simulink model "MatlabBlueprint"  (R2017a)
settings: Solver=VariableStepAuto  StartTime=0.0  StopTime=10.0  RelTol=1e-3
libraries: hdlsllib x25, simulink x1
settings Model: Creator=rafaelmosca  LastModifiedBy=rafaelmosca

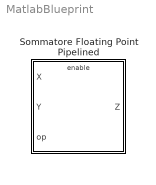
== system MatlabBlueprint ==
  Sommatore Floating Point Pipelined : Subsystem  TreatAsAtomicUnit=on

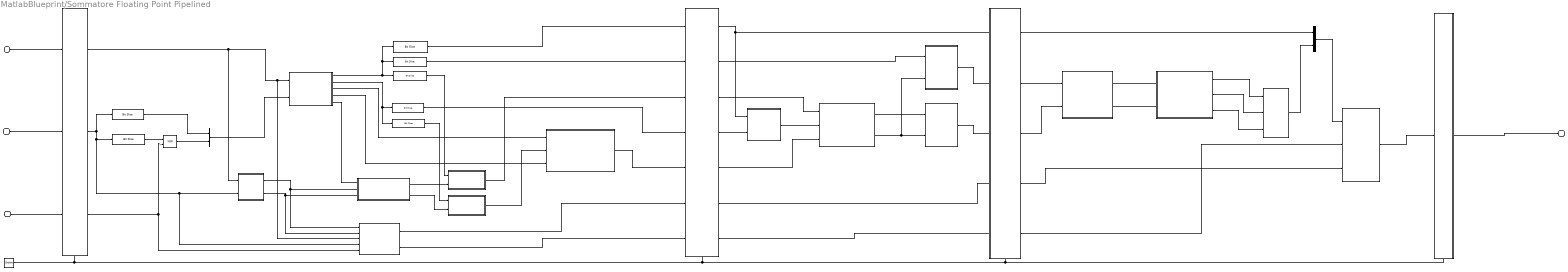
== system MatlabBlueprint/Sommatore Floating Point Pipelined ==
  note: Pre-somma
  note: Somma
  note: Correttiva
  X : Inport
  Y : Inport  Port=2
  op : Inport  Port=3
  clk : EnablePort  ShowOutputPort=on
  "Exp Adjustment " : Subsystem
  ExpChoice : Subsystem
  ExtendG : Subsystem
  ExtendS : Subsystem
  GE : hdlsllib/HDL Operations/Bit Slice  lidx=30  ridx=22
      settings: SourceProductName=HDL Coder  SourceProductBaseCode=HD
  GM : hdlsllib/HDL Operations/Bit Slice  lidx=22  ridx=0
      settings: SourceProductName=HDL Coder  SourceProductBaseCode=HD
  GS : hdlsllib/HDL Operations/Bit Slice  lidx=31  ridx=30
      settings: SourceProductName=HDL Coder  SourceProductBaseCode=HD
  MEY : hdlsllib/HDL Operations/Bit Slice  lidx=30  ridx=0
      settings: SourceProductName=HDL Coder  SourceProductBaseCode=HD
  MUX : Subsystem
  MUX Ris : Subsystem
  "Mantissa Adjustment " : Subsystem
  Normalization Module : Subsystem
  OPlogic : Subsystem
  REG1 : Subsystem  TreatAsAtomicUnit=on
  REG2 : Subsystem  TreatAsAtomicUnit=on
  REGIN : Subsystem  TreatAsAtomicUnit=on
  REGOut : Subsystem  TreatAsAtomicUnit=on
  Rounding : Subsystem
  SM : hdlsllib/HDL Operations/Bit Slice  lidx=22  ridx=0
      settings: SourceProductName=HDL Coder  SourceProductBaseCode=HD
  SS : hdlsllib/HDL Operations/Bit Slice  lidx=31  ridx=30
      settings: SourceProductName=HDL Coder  SourceProductBaseCode=HD
  SY : hdlsllib/HDL Operations/Bit Slice  lidx=31  ridx=30
      settings: SourceProductName=HDL Coder  SourceProductBaseCode=HD
  Shifter : Subsystem
  Somma Mantisse : Subsystem
  "Special Case Handler " : Subsystem
  Special Case Identifier : Subsystem
  Substraction Handling : Concatenate
  Swap : Subsystem  TreatAsAtomicUnit=on
  Vector Concatenate : Concatenate
  XOR : Logic  Operator=XOR  IconShape=distinctive  AllPortsSameDT=off  OutDataTypeStr=boolean
  Z : Outport
  wires:
  X/1 -> REGIN/1(Xin)
  Y/1 -> REGIN/2(Yin)
  clk/1 -> REGIN/Enable, REGOut/Enable, REG2/Enable, REG1/Enable
  op/1 -> REGIN/3(opin)
  REGIN/1(Xout) -> Special Case Identifier/1(X), "Special Case Handler "/3(X), Swap/1(X)
  REGIN/3("opOut ") -> XOR/2, "Special Case Handler "/5(op)
  REG1/7(isSROut) -> REG2/5(isSRin)
  MUX Ris/1(Result) -> REGOut/1(Zin)
  "Special Case Handler "/1(SpecialResult) -> REG1/6("SRin ")
  REGIN/2(Yout) -> MEY/1, SY/1, "Special Case Handler "/4(Y), Special Case Identifier/2(Y)
  GM/1 -> ExtendG/1(MG)
  Swap/1(GreatestNum) -> GS/1, GE/1, GM/1
  Swap/2(SmallestNum) -> SM/1, SS/1
  SM/1 -> ExtendS/1(MS)
  MUX/2(isSSubnormal) -> ExtendS/2(isSSubnormal)
  MUX/1(isGSubnormal) -> ExtendG/2(isGSubnormalG)
  Swap/5(swapped) -> MUX/1(Swapped)
  ExtendS/1("MSE(27) ") -> Shifter/2(Mantissa (27))
  Swap/3(Diff(5)) -> Shifter/1("ShiftNum (5) ")
  ExtendG/1("MGE(27) ") -> REG1/3(GEM)
  GE/1 -> REG1/2(GE)
  GS/1 -> REG1/1(GS)
  SS/1 -> REG1/4(SS)
  Shifter/1(Mantissa Shiftata (27)) -> REG1/5(SEM)
  REG1/3(GEMOut) -> Somma Mantisse/1("G ")
  REG1/5(SEMOut) -> Somma Mantisse/3(S)
  OPlogic/1(AdderOp) -> Somma Mantisse/2(Op)
  REG1/1(GSout) -> OPlogic/1("Segno 1 "), REG2/1(ZS)
  REG1/4(SSOut) -> OPlogic/2(Segno 2)
  REG1/6(SROut 7) -> REG2/4(SRin)
  REG2/5(isSRout) -> MUX Ris/2("isSpecialSR ")
  REG2/4(SRout 7) -> MUX Ris/3(SpecialResult)
  REG2/3(ZEMOut) -> Normalization Module/2("Mantissa ")
  REG2/2(ZEout) -> Normalization Module/1("CurrExp ")
  Normalization Module/1("NormMan ") -> Rounding/1("Mantissa ")
  Rounding/1(EsponenteCorretto(8)) -> ExpChoice/1("CurrExp ")
  Rounding/2("MantissaCorretta(23) ") -> ExpChoice/2(CurrM 1)
  ExpChoice/1(ZEM) -> Vector Concatenate/2
  REG2/1(ZSout) -> Vector Concatenate/1
  Vector Concatenate/1 -> MUX Ris/1(GenereatedResult)
  Swap/4(ForceMZero) -> Shifter/3(ForceMToZero)
  REGOut/1(Zout) -> Z/1
  SY/1 -> XOR/1
  Substraction Handling/1 -> Swap/2(Y)
  Rounding/3(isInfinity) -> ExpChoice/3(isInfinity)
  XOR/1 -> Substraction Handling/2
  MEY/1 -> Substraction Handling/1
  Special Case Identifier/2(CasoY) -> MUX/3(CaseY), "Special Case Handler "/2(CasoY)
  Special Case Identifier/1(CasoX) -> MUX/2(CaseX), "Special Case Handler "/1(CasoX)
  Somma Mantisse/2(AdditionOverflow) -> "Exp Adjustment "/2(Overflow), "Mantissa Adjustment "/2("Overflow ")
  Somma Mantisse/1("MantissaRisultato(27) ") -> "Mantissa Adjustment "/1("Mantissa ")
  "Exp Adjustment "/1(AdjExp) -> REG2/2(ZE)
  REG1/2(GEout) -> "Exp Adjustment "/1("Exp ")
  Normalization Module/2("NExp ") -> Rounding/2(Exponent)
  "Mantissa Adjustment "/1(AdjMant) -> REG2/3(ZEM)
  "Special Case Handler "/2("isSpecialResult ") -> REG1/7(isSR)

== system MatlabBlueprint/Sommatore Floating Point Pipelined/Exp Adjustment  ==
  note: Infinity
  note: Da sistemare quando è infinito
  "Exp " : Inport
  Overflow : Inport  Port=2
  Add : Sum
  Constant1 : Constant  Value=254
  Logical Operator : Logic  IconShape=distinctive  AllPortsSameDT=off  OutDataTypeStr=boolean
  Relational Operator : RelationalOperator  Operator===  OutDataTypeStr=boolean  RndMeth=Simplest
  AdjExp : Outport
  wires:
  "Exp "/1 -> Add/1, Relational Operator/2
  Constant1/1 -> Relational Operator/1
  Relational Operator/1 -> Logical Operator/1
  Overflow/1 -> Add/2, Logical Operator/2
  Logical Operator/1 -> ?
  Add/1 -> AdjExp/1

== system MatlabBlueprint/Sommatore Floating Point Pipelined/ExpChoice ==
  note: Da considerare il bit implicito e quelli di arrotondamento
  "CurrExp " : Inport
  CurrM 1 : Inport  Port=2
  isInfinity : Inport  Port=3
  ZEM : Outport

== system MatlabBlueprint/Sommatore Floating Point Pipelined/ExtendG ==
  MG : Inport
  isGSubnormalG : Inport  Port=2
  Constant : Constant  Value=000
  ImplicitBit : Logic  Operator=NOT  IconShape=distinctive  AllPortsSameDT=off  OutDataTypeStr=boolean
  Vector Concatenate : Concatenate  NumInputs=3
  "MGE(27) " : Outport
  wires:
  Vector Concatenate/1 -> "MGE(27) "/1
  isGSubnormalG/1 -> ImplicitBit/1
  ImplicitBit/1 -> Vector Concatenate/1
  MG/1 -> Vector Concatenate/2
  Constant/1 -> Vector Concatenate/3

== system MatlabBlueprint/Sommatore Floating Point Pipelined/ExtendS ==
  MS : Inport
  isSSubnormal : Inport  Port=2
  Constant : Constant  Value=000
  ImplicitBit : Logic  Operator=NOT  IconShape=distinctive  AllPortsSameDT=off  OutDataTypeStr=boolean
  Vector Concatenate : Concatenate  NumInputs=3
  "MSE(27) " : Outport
  wires:
  Vector Concatenate/1 -> "MSE(27) "/1
  isSSubnormal/1 -> ImplicitBit/1
  MS/1 -> Vector Concatenate/2
  Constant/1 -> Vector Concatenate/3
  ImplicitBit/1 -> Vector Concatenate/1

== system MatlabBlueprint/Sommatore Floating Point Pipelined/MUX ==
  note: if SWAPPED=1 CASO Y becomes CASOG
  Swapped : Inport
  CaseX : Inport  Port=2
  CaseY : Inport  Port=3
  isXSubnormal : hdlsllib/HDL Operations/Bit Slice  lidx=3  ridx=3
      settings: SourceProductName=HDL Coder  SourceProductBaseCode=HD
  isYSubnormal : hdlsllib/HDL Operations/Bit Slice  lidx=3  ridx=3
      settings: SourceProductName=HDL Coder  SourceProductBaseCode=HD
  isGSubnormal : Outport
  isSSubnormal : Outport  Port=2
  wires:
  CaseX/1 -> isXSubnormal/1
  CaseY/1 -> isYSubnormal/1

== system MatlabBlueprint/Sommatore Floating Point Pipelined/MUX Ris ==
  GenereatedResult : Inport
  "isSpecialSR " : Inport  Port=2
  SpecialResult : Inport  Port=3
  Result : Outport
  wires:
  GenereatedResult/1 -> ?

== system MatlabBlueprint/Sommatore Floating Point Pipelined/Mantissa Adjustment  ==
  note: perdo l'ultimo
  note: shift a destra di una posizione per gestire l'overflow
  note: 0
  note: 1
  "Mantissa " : Inport
  "Overflow " : Inport  Port=2
  "       " : hdlsllib/HDL Operations/Bit Slice  lidx=26  ridx=1
      settings: SourceProductName=HDL Coder  SourceProductBaseCode=HD
  Switch : Switch  Criteria=u2 ~= 0
  Vector Concatenate : Concatenate
  AdjMant : Outport
  wires:
  Switch/1 -> AdjMant/1
  "       "/1 -> Vector Concatenate/2
  "Mantissa "/1 -> Switch/1, "       "/1
  "Overflow "/1 -> Vector Concatenate/1, Switch/2
  Vector Concatenate/1 -> Switch/3

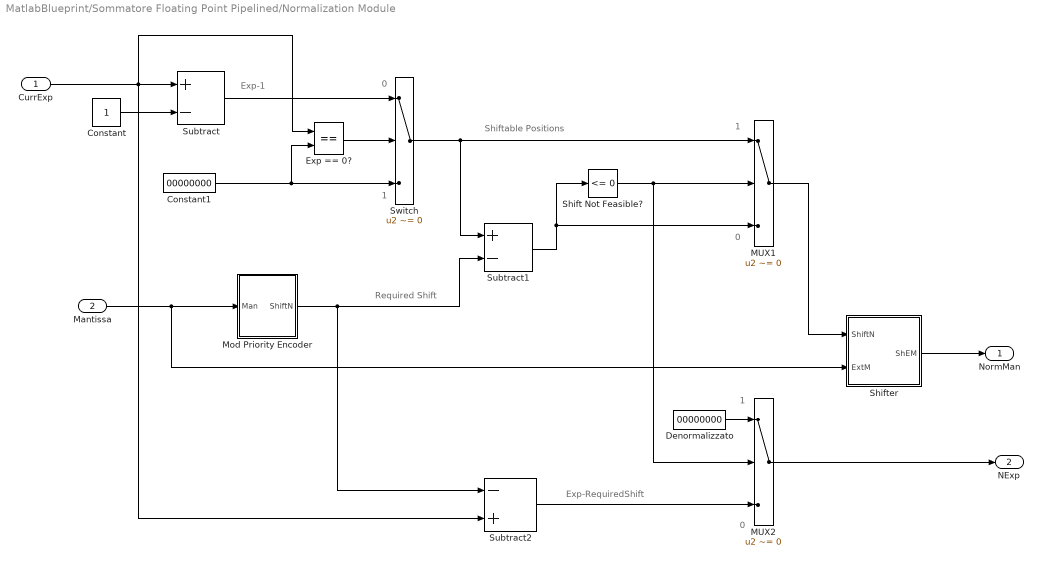
== system MatlabBlueprint/Sommatore Floating Point Pipelined/Normalization Module ==
  note: Exp-1
  note: Exp-RequiredShift
  note: Required Shift
  note: 0
  note: Shiftable Positions
  note: 1
  note: 1
  note: 0
  note: 1
  note: 0
  "CurrExp " : Inport
  "Mantissa " : Inport  Port=2
  Constant : Constant
  Constant1 : Constant  Value=00000000
  Denormalizzato : Constant  Value=00000000
  Exp == 0? : RelationalOperator  Operator===  OutDataTypeStr=boolean  RndMeth=Simplest
  MUX1 : Switch  Criteria=u2 ~= 0
  MUX2 : Switch  Criteria=u2 ~= 0
  "Mod Priority Encoder " : Subsystem
  Shift Not Feasible? : simulink/Logic and Bit Operations/Compare To Zero  relop=<=  OutDataTypeStr=boolean
  Shifter : Subsystem
  Subtract : Sum  Inputs=+-
  Subtract1 : Sum  Inputs=+-
  "Subtract2 " : Sum  Inputs=-+
  Switch : Switch  Criteria=u2 ~= 0
  "NormMan " : Outport
  "NExp " : Outport  Port=2
  wires:
  "Mantissa "/1 -> "Mod Priority Encoder "/1(Man), Shifter/2(ExtM)
  "CurrExp "/1 -> "Subtract2 "/2, Subtract/1, Exp == 0?/1
  "Mod Priority Encoder "/1(ShiftN) -> "Subtract2 "/1, Subtract1/2
  Shifter/1(ShEM) -> "NormMan "/1
  Constant/1 -> Subtract/2
  Subtract/1 -> Switch/1
  Exp == 0?/1 -> Switch/2
  Constant1/1 -> Switch/3, Exp == 0?/2
  Switch/1 -> MUX1/1, Subtract1/1
  MUX1/1 -> Shifter/1("ShiftN ")
  Subtract1/1 -> Shift Not Feasible?/1, MUX1/3
  Shift Not Feasible?/1 -> MUX2/2, MUX1/2
  "Subtract2 "/1 -> MUX2/3
  Denormalizzato/1 -> MUX2/1
  MUX2/1 -> "NExp "/1

== system MatlabBlueprint/Sommatore Floating Point Pipelined/OPlogic ==
  note: Non conta l'ordine!!!!! il segno viene gestit dal numero più grande
  "Segno 1 " : Inport
  Segno 2 : Inport  Port=2
  OpLogic : Logic  Operator=XOR  IconShape=distinctive  AllPortsSameDT=off  OutDataTypeStr=boolean
  AdderOp : Outport
  wires:
  "Segno 1 "/1 -> OpLogic/1
  Segno 2/1 -> OpLogic/2
  OpLogic/1 -> AdderOp/1

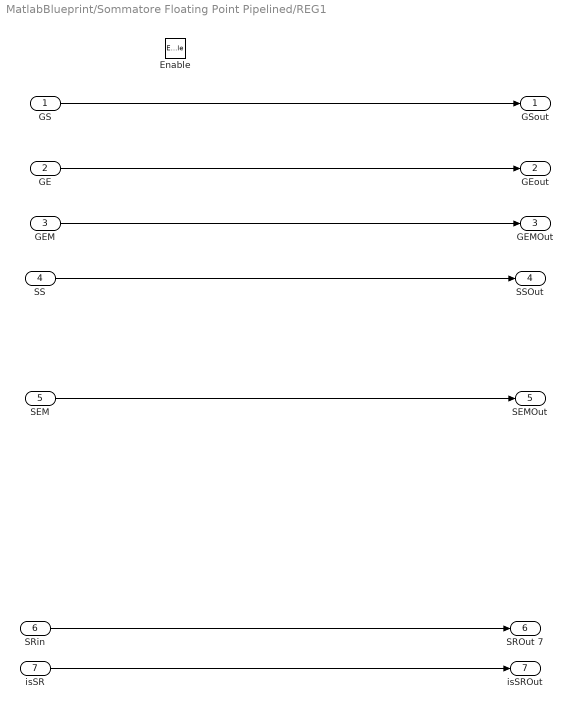
== system MatlabBlueprint/Sommatore Floating Point Pipelined/REG1 ==
  GS : Inport
  GE : Inport  Port=2
  GEM : Inport  Port=3
  SS : Inport  Port=4
  SEM : Inport  Port=5
  "SRin " : Inport  Port=6
  isSR : Inport  Port=7
  Enable : EnablePort
  GSout : Outport
  GEout : Outport  Port=2
  GEMOut : Outport  Port=3
  SSOut : Outport  Port=4
  SEMOut : Outport  Port=5
  SROut 7 : Outport  Port=6
  isSROut : Outport  Port=7
  wires:
  GS/1 -> GSout/1
  GE/1 -> GEout/1
  GEM/1 -> GEMOut/1
  SS/1 -> SSOut/1
  SEM/1 -> SEMOut/1
  "SRin "/1 -> SROut 7/1
  isSR/1 -> isSROut/1

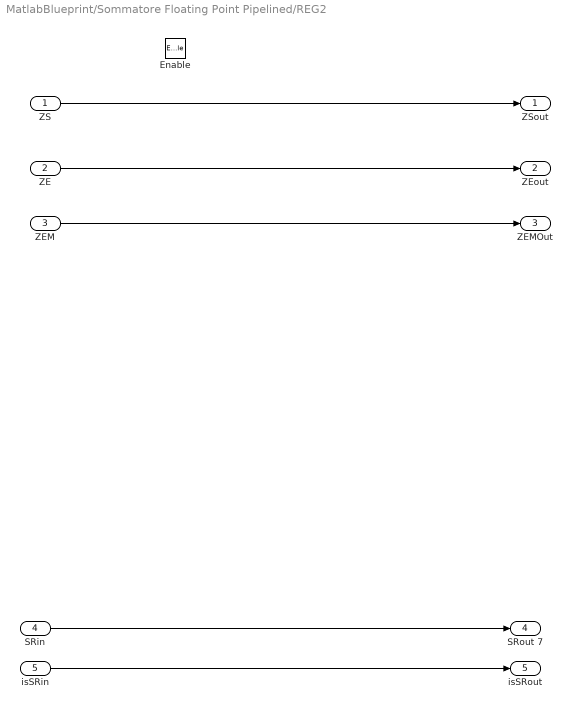
== system MatlabBlueprint/Sommatore Floating Point Pipelined/REG2 ==
  ZS : Inport
  ZE : Inport  Port=2
  ZEM : Inport  Port=3
  SRin : Inport  Port=4
  isSRin : Inport  Port=5
  Enable : EnablePort
  ZSout : Outport
  ZEout : Outport  Port=2
  ZEMOut : Outport  Port=3
  SRout 7 : Outport  Port=4
  isSRout : Outport  Port=5
  wires:
  ZS/1 -> ZSout/1
  ZE/1 -> ZEout/1
  ZEM/1 -> ZEMOut/1
  SRin/1 -> SRout 7/1
  isSRin/1 -> isSRout/1

== system MatlabBlueprint/Sommatore Floating Point Pipelined/REGIN ==
  Xin : Inport
  Yin : Inport  Port=2
  opin : Inport  Port=3
  Enable : EnablePort
  Xout : Outport
  Yout : Outport  Port=2
  "opOut " : Outport  Port=3
  wires:
  Xin/1 -> Xout/1
  Yin/1 -> Yout/1
  opin/1 -> "opOut "/1

== system MatlabBlueprint/Sommatore Floating Point Pipelined/REGOut ==
  Zin : Inport
  Enable : EnablePort
  Zout : Outport
  wires:
  Zin/1 -> Zout/1

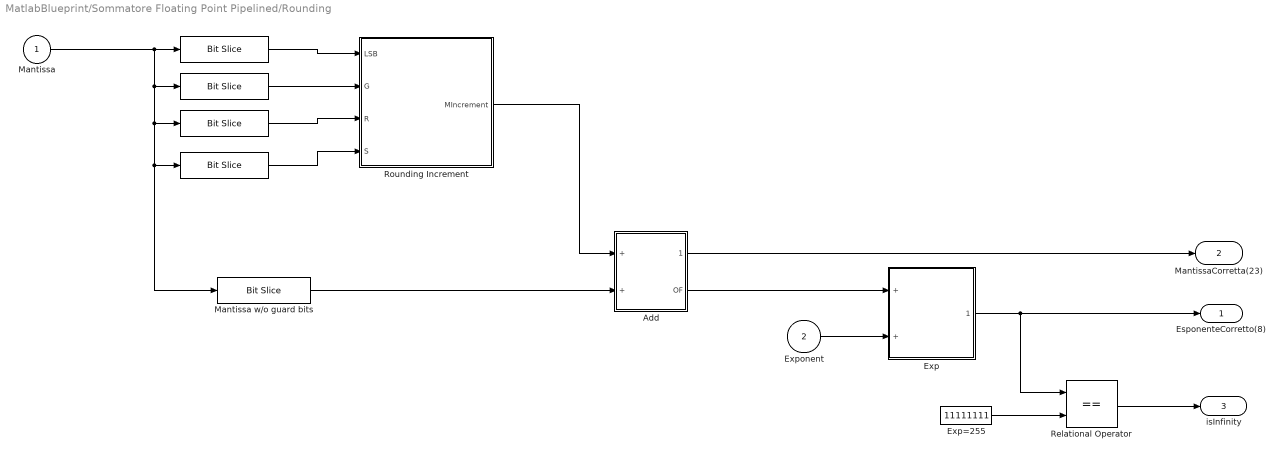
== system MatlabBlueprint/Sommatore Floating Point Pipelined/Rounding ==
  "Mantissa " : Inport
  Exponent : Inport  Port=2
  " " : hdlsllib/HDL Operations/Bit Slice  lidx=3  ridx=3
      settings: SourceProductName=HDL Coder  SourceProductBaseCode=HD
  "  " : hdlsllib/HDL Operations/Bit Slice  lidx=0  ridx=0
      settings: SourceProductName=HDL Coder  SourceProductBaseCode=HD
  "   " : hdlsllib/HDL Operations/Bit Slice  lidx=2  ridx=2
      settings: SourceProductName=HDL Coder  SourceProductBaseCode=HD
  "       " : hdlsllib/HDL Operations/Bit Slice  lidx=1  ridx=1
      settings: SourceProductName=HDL Coder  SourceProductBaseCode=HD
  "  Mantissa w/o guard bits" : hdlsllib/HDL Operations/Bit Slice  lidx=25  ridx=3
      settings: SourceProductName=HDL Coder  SourceProductBaseCode=HD
  Add : Subsystem
  Exp : Subsystem
  Exp=255 : Constant  Value=11111111
  Relational Operator : RelationalOperator  Operator===  OutDataTypeStr=boolean  RndMeth=Simplest
  Rounding Increment : Subsystem
  EsponenteCorretto(8) : Outport
  "MantissaCorretta(23) " : Outport  Port=2
  isInfinity : Outport  Port=3
  wires:
  "Mantissa "/1 -> "  Mantissa w/o guard bits"/1, "  "/1, "       "/1, "   "/1, " "/1
  " "/1 -> Rounding Increment/1("LSB ")
  "   "/1 -> Rounding Increment/2("G ")
  "       "/1 -> Rounding Increment/3(R)
  "  "/1 -> Rounding Increment/4(S)
  Rounding Increment/1("MIncrement ") -> Add/1("+ ")
  "  Mantissa w/o guard bits"/1 -> Add/2("+ ")
  Add/2(" OF") -> Exp/1("+ ")
  Exponent/1 -> Exp/2("+ ")
  Add/1(" ") -> "MantissaCorretta(23) "/1
  Exp/1(" ") -> EsponenteCorretto(8)/1, Relational Operator/1
  Relational Operator/1 -> isInfinity/1
  Exp=255/1 -> Relational Operator/2

== system MatlabBlueprint/Sommatore Floating Point Pipelined/Shifter ==
  "ShiftNum (5) " : Inport
  Mantissa (27) : Inport  Port=2
  ForceMToZero : Inport  Port=3
  Esempio 4 bit : Subsystem
  Mantissa Shiftata (27) : Outport

== system MatlabBlueprint/Sommatore Floating Point Pipelined/Somma Mantisse ==
  note: Da considerare il bit implicito e quelli di arrotondamento
  "G " : Inport
  Op : Inport  Port=2
  S : Inport  Port=3
  "MantissaRisultato(27) " : Outport
  AdditionOverflow : Outport  Port=2

== system MatlabBlueprint/Sommatore Floating Point Pipelined/Special Case Handler  ==
  CasoX : Inport
  CasoY : Inport  Port=2
  X : Inport  Port=3
  Y : Inport  Port=4
  op : Inport  Port=5
  SpecialResult : Outport
  "isSpecialResult " : Outport  Port=2

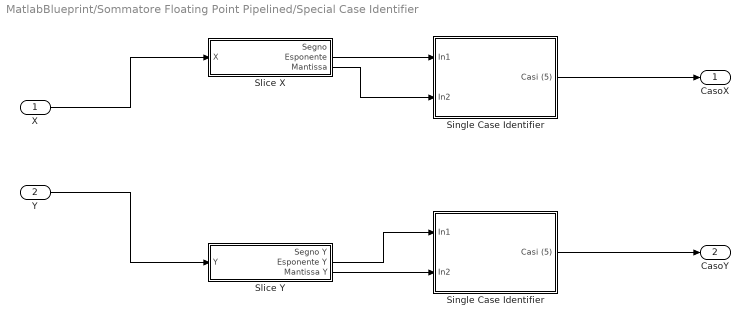
== system MatlabBlueprint/Sommatore Floating Point Pipelined/Special Case Identifier ==
  X : Inport
  Y : Inport  Port=2
  Single Case Identifier : Subsystem
  "Single Case Identifier " : Subsystem
  Slice X : Subsystem
  Slice Y : Subsystem
  CasoX : Outport
  CasoY : Outport  Port=2
  wires:
  Slice Y/3(Mantissa Y) -> "Single Case Identifier "/2(In2)
  Slice X/3(Mantissa) -> Single Case Identifier/2(In2)
  Slice Y/2(Esponente Y) -> "Single Case Identifier "/1(In1)
  Slice X/2(Esponente) -> Single Case Identifier/1(In1)
  X/1 -> Slice X/1("X ")
  Y/1 -> Slice Y/1("Y ")
  Single Case Identifier/1(Casi (5)) -> CasoX/1
  "Single Case Identifier "/1(Casi (5)) -> CasoY/1

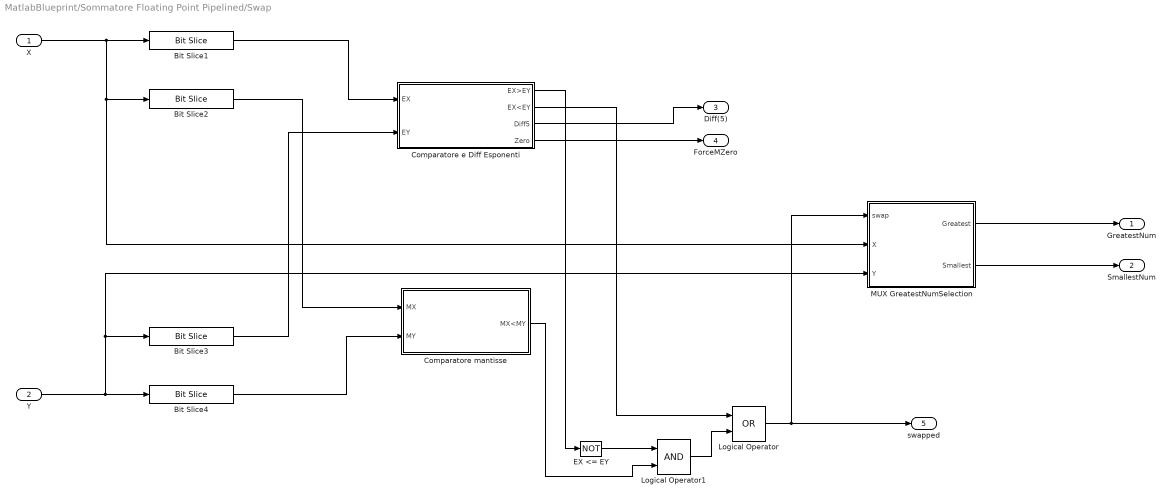
== system MatlabBlueprint/Sommatore Floating Point Pipelined/Swap ==
  X : Inport
  Y : Inport  Port=2
  Bit Slice1 : hdlsllib/HDL Operations/Bit Slice  lidx=30  ridx=22
      settings: SourceProductName=HDL Coder  SourceProductBaseCode=HD
  Bit Slice2 : hdlsllib/HDL Operations/Bit Slice  lidx=22  ridx=0
      settings: SourceProductName=HDL Coder  SourceProductBaseCode=HD
  Bit Slice3 : hdlsllib/HDL Operations/Bit Slice  lidx=30  ridx=22
      settings: SourceProductName=HDL Coder  SourceProductBaseCode=HD
  Bit Slice4 : hdlsllib/HDL Operations/Bit Slice  lidx=22  ridx=0
      settings: SourceProductName=HDL Coder  SourceProductBaseCode=HD
  Comparatore e Diff Esponenti : Subsystem
  Comparatore mantisse : Subsystem
  EX <= EY : Logic  Operator=NOT  IconShape=distinctive  AllPortsSameDT=off  OutDataTypeStr=boolean
  Logical Operator : Logic  Operator=OR  IconShape=distinctive  AllPortsSameDT=off  OutDataTypeStr=boolean
  Logical Operator1 : Logic  IconShape=distinctive  AllPortsSameDT=off  OutDataTypeStr=boolean
  MUX GreatestNumSelection : Subsystem
  GreatestNum : Outport
  SmallestNum : Outport  Port=2
  Diff(5) : Outport  Port=3
  ForceMZero : Outport  Port=4
  swapped : Outport  Port=5
  wires:
  Y/1 -> Bit Slice4/1, MUX GreatestNumSelection/3(Y), Bit Slice3/1
  Bit Slice1/1 -> Comparatore e Diff Esponenti/1(EX)
  Bit Slice3/1 -> Comparatore e Diff Esponenti/2(EY)
  Bit Slice2/1 -> Comparatore mantisse/1(MX)
  Bit Slice4/1 -> Comparatore mantisse/2(MY)
  Comparatore e Diff Esponenti/1(EX>EY) -> EX <= EY/1
  MUX GreatestNumSelection/2("Smallest ") -> SmallestNum/1
  Logical Operator1/1 -> Logical Operator/2
  Logical Operator/1 -> swapped/1, MUX GreatestNumSelection/1("swap ")
  X/1 -> Bit Slice1/1, MUX GreatestNumSelection/2(X), Bit Slice2/1
  Comparatore e Diff Esponenti/2(EX<EY) -> Logical Operator/1
  Comparatore mantisse/1(MX<MY) -> Logical Operator1/2
  EX <= EY/1 -> Logical Operator1/1
  MUX GreatestNumSelection/1(Greatest) -> GreatestNum/1
  Comparatore e Diff Esponenti/3(Diff5) -> Diff(5)/1
  Comparatore e Diff Esponenti/4(Zero) -> ForceMZero/1

== system MatlabBlueprint/Sommatore Floating Point Pipelined/Normalization Module/Mod Priority Encoder  ==
  note: 5 bit
  Man : Inport
  ShiftN : Outport

== system MatlabBlueprint/Sommatore Floating Point Pipelined/Normalization Module/Shifter ==
  "ShiftN " : Inport
  ExtM : Inport  Port=2
  ShEM : Outport

== system MatlabBlueprint/Sommatore Floating Point Pipelined/Rounding/Add ==
  "+ " : Inport
  "+ " : Inport  Port=2
  " " : Outport
  " OF" : Outport  Port=2

== system MatlabBlueprint/Sommatore Floating Point Pipelined/Rounding/Exp ==
  "+ " : Inport
  "+ " : Inport  Port=2
  " " : Outport

== system MatlabBlueprint/Sommatore Floating Point Pipelined/Rounding/Rounding Increment ==
  "LSB " : Inport
  "G " : Inport  Port=2
  R : Inport  Port=3
  S : Inport  Port=4
  "MIncrement " : Outport

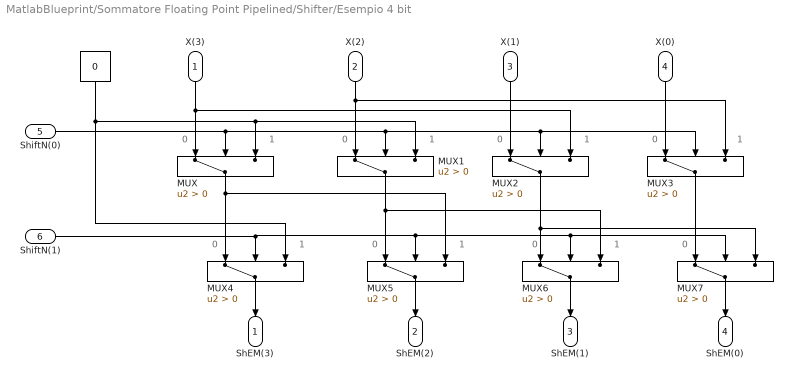
== system MatlabBlueprint/Sommatore Floating Point Pipelined/Shifter/Esempio 4 bit ==
  note: 0
  note: 1
  note: 1
  note: 0
  note: 0
  note: 0
  note: 0
  note: 1
  note: 0
  note: 1
  note: 1
  note: 1
  note: 0
  note: 0
  note: 1
  X(3) : Inport
  X(2) : Inport  Port=2
  X(1) : Inport  Port=3
  X(0) : Inport  Port=4
  ShiftN(0) : Inport  Port=5
  ShiftN(1) : Inport  Port=6
  " " : Constant  Value=0
  MUX{,1..7} (8 alike) : Switch  Criteria=u2 > Threshold
  ShEM(3) : Outport
  ShEM(2) : Outport  Port=2
  ShEM(1) : Outport  Port=3
  ShEM(0) : Outport  Port=4
  wires:
  MUX2/1 -> MUX7/3, MUX6/1
  X(1)/1 -> MUX2/1
  ShiftN(0)/1 -> MUX/2, MUX1/2, MUX2/2, MUX3/2
  X(2)/1 -> MUX1/1, MUX3/3
  MUX/1 -> MUX4/1, MUX5/3
  " "/1 -> MUX4/3, MUX/3, MUX1/3
  MUX4/1 -> ShEM(3)/1
  MUX5/1 -> ShEM(2)/1
  X(0)/1 -> MUX3/1
  MUX3/1 -> MUX7/1
  X(3)/1 -> MUX/1, MUX2/3
  MUX6/1 -> ShEM(1)/1
  ShiftN(1)/1 -> MUX5/2, MUX6/2, MUX7/2, MUX4/2
  MUX1/1 -> MUX6/3, MUX5/1
  MUX7/1 -> ShEM(0)/1

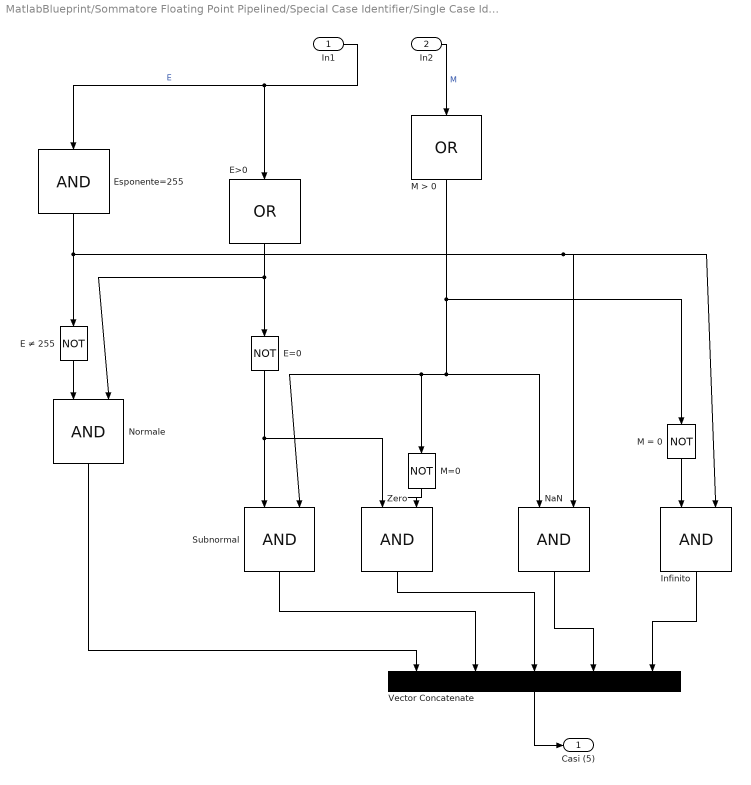
== system MatlabBlueprint/Sommatore Floating Point Pipelined/Special Case Identifier/Single Case Identifier ==
  In1 : Inport
  In2 : Inport  Port=2
  E ≠ 255 : Logic  Operator=NOT  Inputs=1  IconShape=distinctive  AllPortsSameDT=off  OutDataTypeStr=boolean
  E=0 : Logic  Operator=NOT  Inputs=1  IconShape=distinctive  AllPortsSameDT=off  OutDataTypeStr=boolean
  E>0 : Logic  Operator=OR  Inputs=1  IconShape=distinctive  AllPortsSameDT=off  OutDataTypeStr=boolean
  Esponente=255 : Logic  Inputs=1  IconShape=distinctive  AllPortsSameDT=off  OutDataTypeStr=boolean
  Infinito : Logic  IconShape=distinctive  AllPortsSameDT=off  OutDataTypeStr=boolean
  M = 0 : Logic  Operator=NOT  Inputs=1  IconShape=distinctive  AllPortsSameDT=off  OutDataTypeStr=boolean
  M > 0 : Logic  Operator=OR  Inputs=1  IconShape=distinctive  AllPortsSameDT=off  OutDataTypeStr=boolean
  M=0 : Logic  Operator=NOT  Inputs=1  IconShape=distinctive  AllPortsSameDT=off  OutDataTypeStr=boolean
  NaN : Logic  IconShape=distinctive  AllPortsSameDT=off  OutDataTypeStr=boolean
  Normale : Logic  IconShape=distinctive  AllPortsSameDT=off  OutDataTypeStr=boolean
  Subnormal : Logic  IconShape=distinctive  AllPortsSameDT=off  OutDataTypeStr=boolean
  Vector Concatenate : Concatenate  NumInputs=5
  Zero : Logic  IconShape=distinctive  AllPortsSameDT=off  OutDataTypeStr=boolean
  Casi (5) : Outport
  wires:
  Vector Concatenate/1 -> Casi (5)/1
  Normale/1 -> Vector Concatenate/1
  M = 0/1 -> Infinito/1
  NaN/1 -> Vector Concatenate/4
  M=0/1 -> Zero/2
  Subnormal/1 -> Vector Concatenate/2
  E=0/1 -> Zero/1, Subnormal/1
  In2/1 -> M > 0/1  "M"
  Infinito/1 -> Vector Concatenate/5
  E>0/1 -> Normale/2, E=0/1
  In1/1 -> E>0/1, Esponente=255/1  "E"
  M > 0/1 -> M = 0/1, NaN/1, M=0/1, Subnormal/2
  Zero/1 -> Vector Concatenate/3
  Esponente=255/1 -> E ≠ 255/1, Infinito/2, NaN/2
  E ≠ 255/1 -> Normale/1

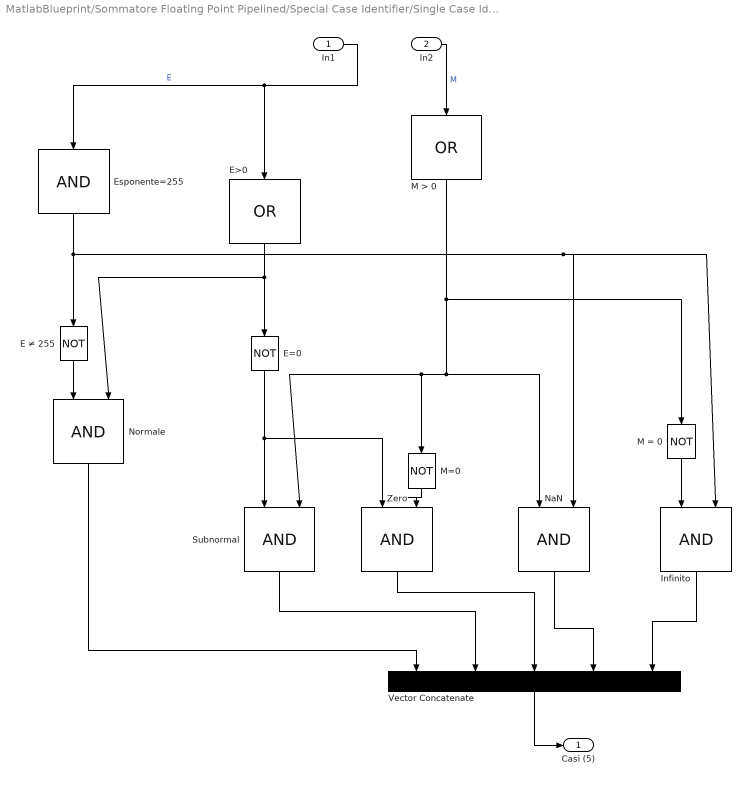
== system MatlabBlueprint/Sommatore Floating Point Pipelined/Special Case Identifier/Single Case Identifier  ==
  In1 : Inport
  In2 : Inport  Port=2
  E ≠ 255 : Logic  Operator=NOT  Inputs=1  IconShape=distinctive  AllPortsSameDT=off  OutDataTypeStr=boolean
  E=0 : Logic  Operator=NOT  Inputs=1  IconShape=distinctive  AllPortsSameDT=off  OutDataTypeStr=boolean
  E>0 : Logic  Operator=OR  Inputs=1  IconShape=distinctive  AllPortsSameDT=off  OutDataTypeStr=boolean
  Esponente=255 : Logic  Inputs=1  IconShape=distinctive  AllPortsSameDT=off  OutDataTypeStr=boolean
  Infinito : Logic  IconShape=distinctive  AllPortsSameDT=off  OutDataTypeStr=boolean
  M = 0 : Logic  Operator=NOT  Inputs=1  IconShape=distinctive  AllPortsSameDT=off  OutDataTypeStr=boolean
  M > 0 : Logic  Operator=OR  Inputs=1  IconShape=distinctive  AllPortsSameDT=off  OutDataTypeStr=boolean
  M=0 : Logic  Operator=NOT  Inputs=1  IconShape=distinctive  AllPortsSameDT=off  OutDataTypeStr=boolean
  NaN : Logic  IconShape=distinctive  AllPortsSameDT=off  OutDataTypeStr=boolean
  Normale : Logic  IconShape=distinctive  AllPortsSameDT=off  OutDataTypeStr=boolean
  Subnormal : Logic  IconShape=distinctive  AllPortsSameDT=off  OutDataTypeStr=boolean
  Vector Concatenate : Concatenate  NumInputs=5
  Zero : Logic  IconShape=distinctive  AllPortsSameDT=off  OutDataTypeStr=boolean
  Casi (5) : Outport
  wires:
  E>0/1 -> Normale/2, E=0/1
  Subnormal/1 -> Vector Concatenate/2
  NaN/1 -> Vector Concatenate/4
  E=0/1 -> Zero/1, Subnormal/1
  Normale/1 -> Vector Concatenate/1
  In2/1 -> M > 0/1  "M"
  Infinito/1 -> Vector Concatenate/5
  Vector Concatenate/1 -> Casi (5)/1
  M = 0/1 -> Infinito/1
  In1/1 -> E>0/1, Esponente=255/1  "E"
  M=0/1 -> Zero/2
  M > 0/1 -> M = 0/1, NaN/1, M=0/1, Subnormal/2
  Zero/1 -> Vector Concatenate/3
  Esponente=255/1 -> E ≠ 255/1, Infinito/2, NaN/2
  E ≠ 255/1 -> Normale/1

== system MatlabBlueprint/Sommatore Floating Point Pipelined/Special Case Identifier/Slice X ==
  "X " : Inport
  Esponente X : hdlsllib/HDL Operations/Bit Slice  lidx=30  ridx=22
      settings: SourceProductName=HDL Coder  SourceProductBaseCode=HD
  Mantissa X : hdlsllib/HDL Operations/Bit Slice  lidx=22  ridx=0
      settings: SourceProductName=HDL Coder  SourceProductBaseCode=HD
  "Segno X " : hdlsllib/HDL Operations/Bit Slice  lidx=31  ridx=30
      settings: SourceProductName=HDL Coder  SourceProductBaseCode=HD
  Segno : Outport
  Esponente : Outport  Port=2
  Mantissa : Outport  Port=3
  wires:
  "Segno X "/1 -> Segno/1
  "X "/1 -> Mantissa X/1, Esponente X/1, "Segno X "/1
  Esponente X/1 -> Esponente/1
  Mantissa X/1 -> Mantissa/1

== system MatlabBlueprint/Sommatore Floating Point Pipelined/Special Case Identifier/Slice Y ==
  "Y " : Inport
  Esponente X : hdlsllib/HDL Operations/Bit Slice  lidx=30  ridx=22
      settings: SourceProductName=HDL Coder  SourceProductBaseCode=HD
  Mantissa X : hdlsllib/HDL Operations/Bit Slice  lidx=22  ridx=0
      settings: SourceProductName=HDL Coder  SourceProductBaseCode=HD
  "Segno X " : hdlsllib/HDL Operations/Bit Slice  lidx=31  ridx=30
      settings: SourceProductName=HDL Coder  SourceProductBaseCode=HD
  Segno Y : Outport
  Esponente Y : Outport  Port=2
  Mantissa Y : Outport  Port=3
  wires:
  "Segno X "/1 -> Segno Y/1
  "Y "/1 -> Mantissa X/1, Esponente X/1, "Segno X "/1
  Esponente X/1 -> Esponente Y/1
  Mantissa X/1 -> Mantissa Y/1

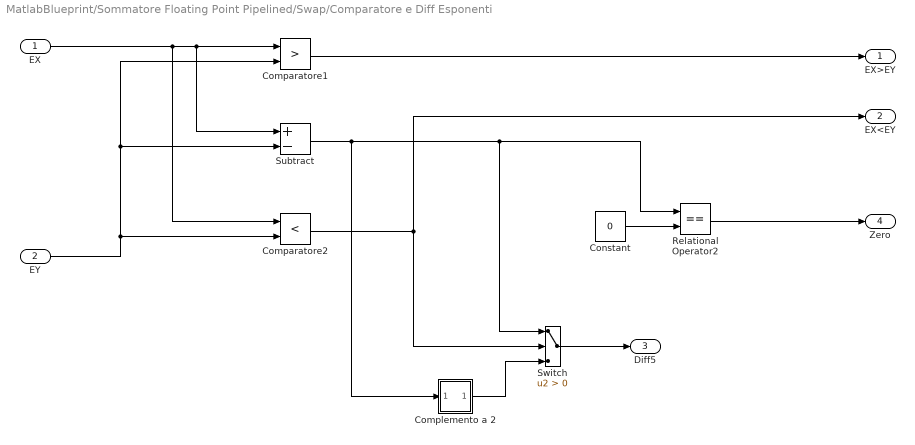
== system MatlabBlueprint/Sommatore Floating Point Pipelined/Swap/Comparatore e Diff Esponenti ==
  EX : Inport
  EY : Inport  Port=2
  Comparatore1 : RelationalOperator  Operator=>  OutDataTypeStr=boolean  RndMeth=Nearest
  Comparatore2 : RelationalOperator  Operator=<  OutDataTypeStr=boolean  RndMeth=Nearest
  Complemento a 2 : Subsystem
  Constant : Constant  Value=0
  Relational Operator2 : RelationalOperator  Operator===  OutDataTypeStr=boolean  RndMeth=Nearest
  Subtract : Sum  Inputs=+-
  Switch : Switch  Criteria=u2 > Threshold
  EX>EY : Outport
  EX<EY : Outport  Port=2
  Diff5 : Outport  Port=3
  Zero : Outport  Port=4  OutDataTypeStr=boolean
  wires:
  EX/1 -> Comparatore2/1, Subtract/1, Comparatore1/1
  EY/1 -> Comparatore2/2, Subtract/2, Comparatore1/2
  Comparatore1/1 -> EX>EY/1
  Subtract/1 -> Complemento a 2/1("in "), Switch/1, Relational Operator2/1
  Constant/1 -> Relational Operator2/2
  Relational Operator2/1 -> Zero/1
  Switch/1 -> Diff5/1
  Comparatore2/1 -> Switch/2, EX<EY/1
  Complemento a 2/1(C2) -> Switch/3

== system MatlabBlueprint/Sommatore Floating Point Pipelined/Swap/Comparatore mantisse ==
  MX : Inport
  MY : Inport  Port=2
  Relational Operator : RelationalOperator  Operator=>  OutDataTypeStr=boolean  RndMeth=Nearest
  MX<MY : Outport
  wires:
  MX/1 -> Relational Operator/1
  MY/1 -> Relational Operator/2
  Relational Operator/1 -> MX<MY/1

== system MatlabBlueprint/Sommatore Floating Point Pipelined/Swap/MUX GreatestNumSelection ==
  note: Se EX>EY MX mantissa numero più grande
      | Se EX<EY MY mantissa numero più grande
      | Se EX=EY e MX >MY MX mantissa numero più grande
      | Se EX=EY e MX<= MY MY mantissa numero più grande
  "swap " : Inport
  X : Inport  Port=2
  Y : Inport  Port=3
  Greatest : Outport
  "Smallest " : Outport  Port=2

== system MatlabBlueprint/Sommatore Floating Point Pipelined/Swap/Comparatore e Diff Esponenti/Complemento a 2 ==
  "in " : Inport
  C2 : Outport
